simulink model "TClabsim2016"  (R2026a)
settings: Solver=VariableStepAuto  StopTime=600
StopFcn:
  | reset_temp
values from neighbouring files (symbols this model uses):
  hlevel = 50    [CA1.m]
settings Model: Creator=jamess  LastModifiedBy=socks

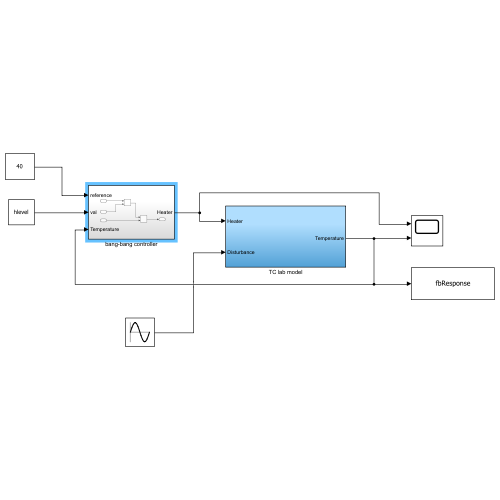
[thumbnail: Simulink's stored preview of the top-level diagram]
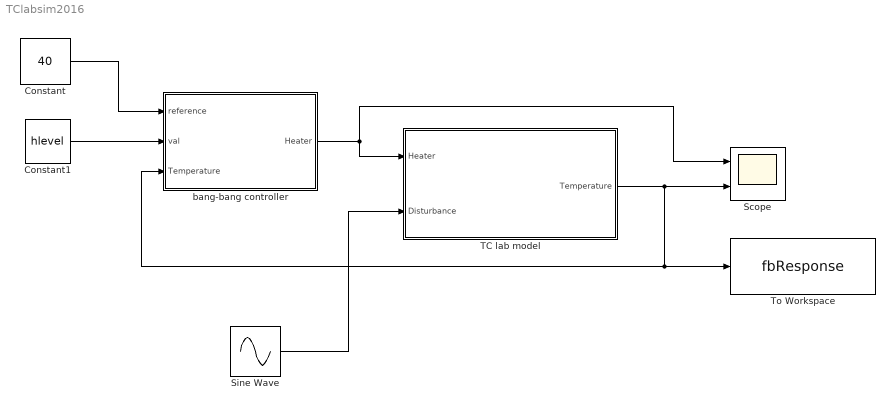
== system TClabsim2016 ==
  Constant : Constant  Value=40
  Constant1 : Constant  Value=hlevel
  Scope : Scope  NumInputPorts=2
      settings: ActiveDisplayYMinimum=20.25  ActiveDisplayYMaximum=37.75
  Sine Wave : Sin  Amplitude=0  Frequency=0  SampleTime=0
  TC lab model : Subsystem
  To Workspace : ToWorkspace  VariableName=fbResponse  SaveFormat=Timeseries  SampleTime=-1
  bang-bang controller : Subsystem
  wires:
  Sine Wave/1 -> TC lab model/2(Disturbance)
  TC lab model/1(Temperature) -> To Workspace/1, bang-bang controller/3(Temperature), Scope/2
  bang-bang controller/1(Heater) -> Scope/1, TC lab model/1(Heater)
  Constant/1 -> bang-bang controller/1(reference)
  Constant1/1 -> bang-bang controller/2(val)

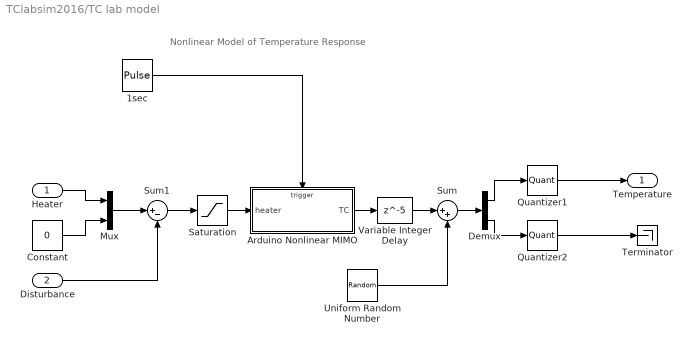
== system TClabsim2016/TC lab model ==
  note: Nonlinear Model of Temperature Response
  Heater : Inport
  Disturbance : Inport  Port=2
  1sec : DiscretePulseGenerator  PulseType=Time based  Period=1  PulseWidth=50
  Arduino Nonlinear MIMO : Subsystem  TreatAsAtomicUnit=on
  Constant : Constant  Value=0
  Demux : Demux  Outputs=2
  Mux : Mux  Inputs=2
  Quantizer1 : Quantizer
  Quantizer2 : Quantizer
  Saturation : Saturate  UpperLimit=100  LowerLimit=0
  Sum : Sum  Inputs=|++
  Sum1 : Sum  Inputs=|+-
  Terminator : Terminator
  Uniform Random Number : UniformRandomNumber  Minimum=[-1;-1]  Maximum=[1;1]  SampleTime=1
  Variable Integer Delay : Delay  DelayLength=5  InitialCondition=23  SampleTime=1
  Temperature : Outport
  wires:
  1sec/1 -> Arduino Nonlinear MIMO/Trigger
  Heater/1 -> Mux/1
  Demux/1 -> Quantizer1/1
  Demux/2 -> Quantizer2/1
  Quantizer1/1 -> Temperature/1
  Quantizer2/1 -> Terminator/1
  Arduino Nonlinear MIMO/1(TC) -> Variable Integer Delay/1
  Uniform Random Number/1 -> Sum/2
  Sum/1 -> Demux/1
  Variable Integer Delay/1 -> Sum/1
  Constant/1 -> Mux/2
  Mux/1 -> Sum1/1
  Disturbance/1 -> Sum1/2
  Saturation/1 -> Arduino Nonlinear MIMO/1(heater)
  Sum1/1 -> Saturation/1

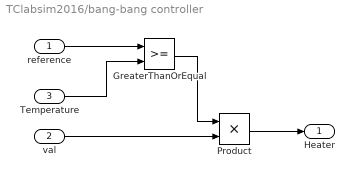
== system TClabsim2016/bang-bang controller ==
  reference : Inport
  val : Inport  Port=2
  Temperature : Inport  Port=3
  GreaterThanOrEqual : RelationalOperator  OutDataTypeStr=boolean  RndMeth=Simplest  InputSameDT=off
  Product : Product
  Heater : Outport
  wires:
  reference/1 -> GreaterThanOrEqual/1
  Temperature/1 -> GreaterThanOrEqual/2
  val/1 -> Product/2
  GreaterThanOrEqual/1 -> Product/1
  Product/1 -> Heater/1

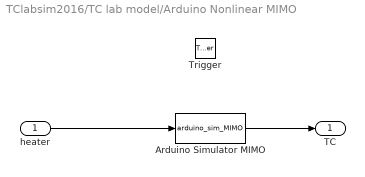
== system TClabsim2016/TC lab model/Arduino Nonlinear MIMO ==
  heater : Inport
  Trigger : TriggerPort  VariantControl=Variant
  Arduino Simulator MIMO : MATLABFcn  MATLABFcn=arduino_sim_MIMO
  TC : Outport  InitialOutput=23
  wires:
  Arduino Simulator MIMO/1 -> TC/1
  heater/1 -> Arduino Simulator MIMO/1
